simulink model "th_duty_cycle_waveform_generator"  (R2020b)
settings: Solver=FixedStepAuto  StartTime=0.0  StopTime=10.0  FixedStep=6.25e-6  RelTol=1e-3
values from neighbouring files (symbols this model uses):
  parOmodFact = 1.0    [dd_model_under_test_data.sldd]
  th_parOutp1TestTol = 0.01    [dd_test_harness_data.sldd]
  th_parOutp2TestTol = 0.0001    [dd_test_harness_data.sldd]
  th_parPWMMode = 4.0    [dd_test_harness_data.sldd]
  th_parSimModeFlag = 0    [dd_test_harness_data.sldd]
libraries: simulink x2
settings Model: DataDictionary=dd_test_harness_data.sldd  EnableAccessToBaseWorkspace=off  PauseTimes=1  Creator=CAV2OFO  LastModifiedBy=CAV2OFO
settings DebuggingCC: ParameterPrecisionLossMsg=none

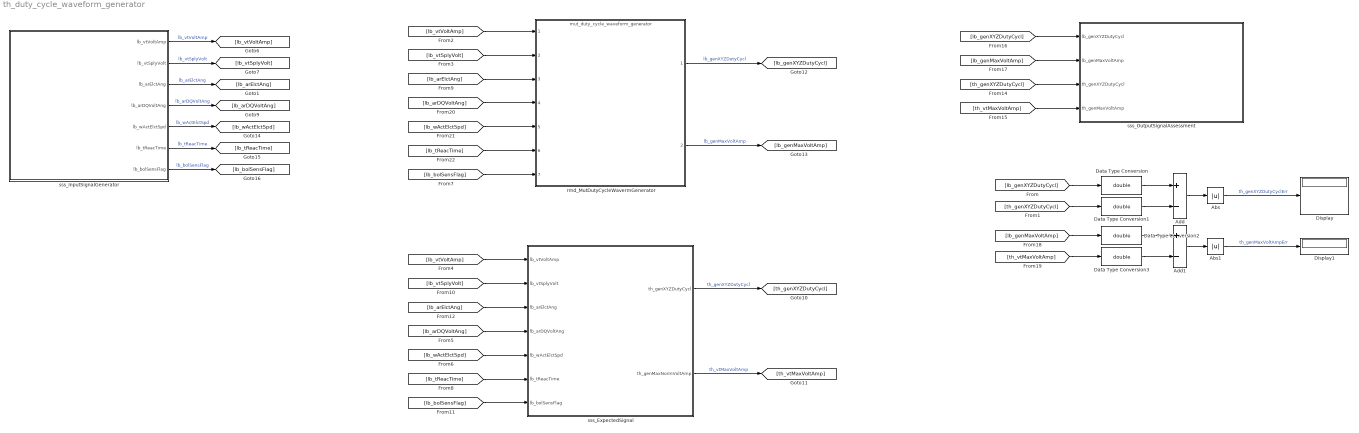
== system th_duty_cycle_waveform_generator ==
  Abs : Abs
  Abs1 : Abs
  Add : Sum  Inputs=+-  OutDataTypeStr=double
  Add1 : Sum  Inputs=+-  OutDataTypeStr=double
  Data Type Conversion{,1..3} (4 alike) : DataTypeConversion  OutDataTypeStr=double
  Display : Display
  Display1 : Display
  rmd_MutDutyCycleWavermGenerator : ModelReference  ModelNameDialog=mut_duty_cycle_waveform_generator  SimulationMode=Normal  ModelReferenceVersion=1.54
  sss_ExpectedSignal : Subsystem
  sss_InputSignalGenerator : Subsystem  InitFcn=|
      | Simulink.suppressDiagnostic([gcb,'/Data Type Conversion1'],...
      |  'SimulinkFixedPoint:util:Overflowoccurred');
      | Simulink.suppressDiagnostic([gcb,'/Data Type Conversion2'],...
      |  'SimulinkFixedPoint:util:Overflowoccurred');
  sss_OutputSignalAssessment : Subsystem
  wires:
  rmd_MutDutyCycleWavermGenerator/1 -> [lb_genXYZDutyCycl]  "lb_genXYZDutyCycl"
  rmd_MutDutyCycleWavermGenerator/2 -> [lb_genMaxVoltAmp]  "lb_genMaxVoltAmp"
  sss_ExpectedSignal/1(th_genXYZDutyCycl) -> [th_genXYZDutyCycl]  "th_genXYZDutyCycl"
  [lb_genXYZDutyCycl] -> Data Type Conversion/1
  [th_genXYZDutyCycl] -> Data Type Conversion1/1
  [lb_genXYZDutyCycl] -> sss_OutputSignalAssessment/1(lb_genXYZDutyCycl)
  Add1/1 -> Abs1/1
  Add/1 -> Abs/1
  Data Type Conversion1/1 -> Add/2
  Data Type Conversion3/1 -> Add1/2
  [th_genXYZDutyCycl] -> sss_OutputSignalAssessment/3(th_genXYZDutyCycl)
  [th_vtMaxVoltAmp] -> sss_OutputSignalAssessment/4(th_genMaxVoltAmp)
  sss_ExpectedSignal/2(th_genMaxNormVoltAmp) -> [th_vtMaxVoltAmp]  "th_vtMaxVoltAmp"
  [th_vtMaxVoltAmp] -> Data Type Conversion3/1
  Data Type Conversion/1 -> Add/1
  Data Type Conversion2/1 -> Add1/1
  Abs1/1 -> Display1/1  "th_genMaxVoltAmpErr"
  [lb_genMaxVoltAmp] -> sss_OutputSignalAssessment/2(lb_genMaxVoltAmp)
  [lb_genMaxVoltAmp] -> Data Type Conversion2/1
  Abs/1 -> Display/1  "th_genXYZDutyCyclErr"
  [lb_vtVoltAmp] -> rmd_MutDutyCycleWavermGenerator/1
  [lb_vtSplyVolt] -> rmd_MutDutyCycleWavermGenerator/2
  [lb_arElctAng] -> rmd_MutDutyCycleWavermGenerator/3
  [lb_arDQVoltAng] -> rmd_MutDutyCycleWavermGenerator/4
  [lb_wActElctSpd] -> rmd_MutDutyCycleWavermGenerator/5
  [lb_tReacTime] -> rmd_MutDutyCycleWavermGenerator/6
  [lb_bolSensFlag] -> rmd_MutDutyCycleWavermGenerator/7
  sss_InputSignalGenerator/1(lb_vtVoltAmp) -> [lb_vtVoltAmp]  "lb_vtVoltAmp"
  sss_InputSignalGenerator/2(lb_vtSplyVolt) -> [lb_vtSplyVolt]  "lb_vtSplyVolt"
  sss_InputSignalGenerator/3(lb_arElctAng) -> [lb_arElctAng]  "lb_arElctAng"
  sss_InputSignalGenerator/4(lb_arDQVoltAng) -> [lb_arDQVoltAng]  "lb_arDQVoltAng"
  sss_InputSignalGenerator/5(lb_wActElctSpd) -> [lb_wActElctSpd]  "lb_wActElctSpd"
  sss_InputSignalGenerator/6(lb_tReacTime) -> [lb_tReacTime]  "lb_tReacTime"
  sss_InputSignalGenerator/7(lb_bolSensFlag) -> [lb_bolSensFlag]  "lb_bolSensFlag"
  [lb_vtVoltAmp] -> sss_ExpectedSignal/1(lb_vtVoltAmp)
  [lb_vtSplyVolt] -> sss_ExpectedSignal/2(lb_vtSplyVolt)
  [lb_arElctAng] -> sss_ExpectedSignal/3(lb_arElctAng)
  [lb_arDQVoltAng] -> sss_ExpectedSignal/4(lb_arDQVoltAng)
  [lb_wActElctSpd] -> sss_ExpectedSignal/5(lb_wActElctSpd)
  [lb_tReacTime] -> sss_ExpectedSignal/6(lb_tReacTime)
  [lb_bolSensFlag] -> sss_ExpectedSignal/7(lb_bolSensFlag)

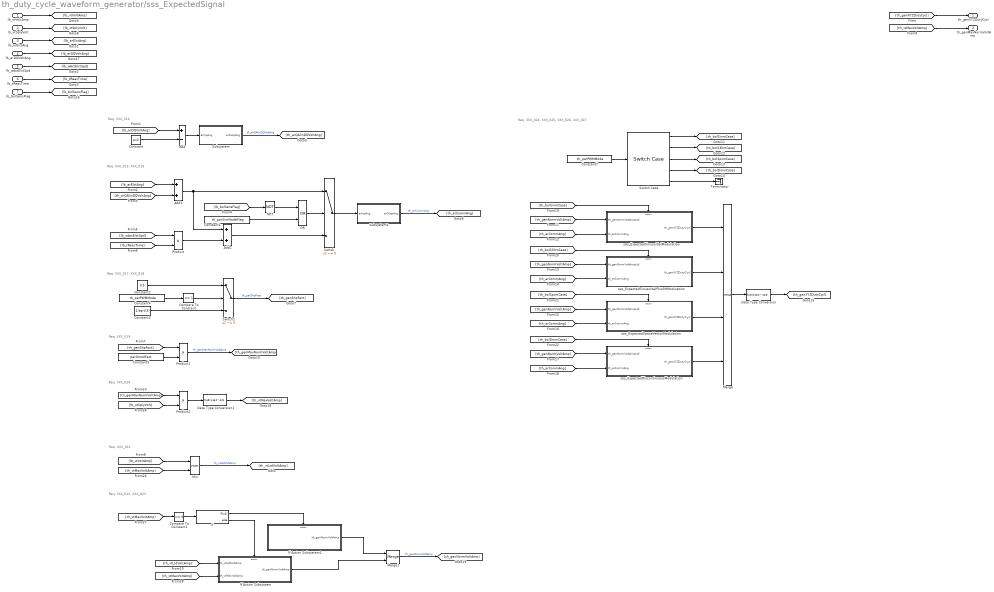
== system th_duty_cycle_waveform_generator/sss_ExpectedSignal ==
  note: Req. XXX_024, XXX_025, XXX_026, XXX_027
  note: Req. XXX_021
  note: Req. XXX_019
  note: Req. XXX_017, XXX_018
  note: Req. XXX_015, XXX_016
  note: Req. XXX_014
  note: Req. XXX_020
  note: Req. XXX_022, XXX_023
  lb_vtVoltAmp : Inport  Interpolate=off
  lb_vtSplyVolt : Inport  Port=2  Interpolate=off
  lb_arElctAng : Inport  Port=3  OutDataTypeStr=fixdt(0,16,pi*2^-15,0)  Interpolate=off
  lb_arDQVoltAng : Inport  Port=4  OutDataTypeStr=fixdt(0,16,pi*2^-15,0)  Interpolate=off
  lb_wActElctSpd : Inport  Port=5  Interpolate=off
  lb_tReacTime : Inport  Port=6  Interpolate=off
  lb_bolSensFlag : Inport  Port=7  OutDataTypeStr=boolean
  Add : Sum  Inputs=+-
  Add1 : Sum
  Add2 : Sum
  Compare To Constant : simulink/Logic and Bit Operations/Compare To Constant  relop===  const=1  OutDataTypeStr=boolean
  Compare To Constant1 : simulink/Logic and Bit Operations/Compare To Constant  relop===  const=0  OutDataTypeStr=boolean
  Constant : Constant  Value=pi/2
  Constant1 : Constant  Value=th_parSimModeFlag
  Constant2 : Constant  Value=0.5
  Constant3 : Constant  Value=1/sqrt(3)
  Constant4 : Constant  Value=th_parPWMMode
  Constant5 : Constant  Value=parOmodFact
  Constant7 : Constant  Value=th_parPWMMode
  Data Type Conversion : DataTypeConversion  OutDataTypeStr=fixdt(0,16,2^-15,0)
  Data Type Conversion1 : DataTypeConversion  OutDataTypeStr=fixdt(1,16,2^-9,0)
  If : If  IfExpression=u1
  If Action Subsystem : Subsystem  TreatAsAtomicUnit=on
  If Action Subsystem1 : Subsystem  TreatAsAtomicUnit=on
  Merge : Merge  Inputs=4
  Merge1 : Merge
  Min : MinMax  Inputs=2
  NOT : Logic  Operator=NOT  IconShape=distinctive  AllPortsSameDT=off  OutDataTypeStr=boolean
  OR : Logic  Operator=OR  AllPortsSameDT=off  OutDataTypeStr=boolean
  Product : Product
  Product1 : Product
  Product2 : Product  OutDataTypeStr=Inherit: Inherit via back propagation
  Subsystem : Subsystem
  Subsystem1 : Subsystem
  Switch : Switch  Criteria=u2 ~= 0
  Switch Case : SwitchCase  CaseConditions={1,2,3,4}
  Switch1 : Switch  Criteria=u2 ~= 0
  Terminator : Terminator
  sas_ExpectedDiscontinuousModulation : Subsystem  TreatAsAtomicUnit=on
  sas_ExpectedSinusoidalModulation : Subsystem  TreatAsAtomicUnit=on
  sas_ExpectedSinusoidalPlus3HModulation : Subsystem  TreatAsAtomicUnit=on
  sas_ExpectedSpaceVectorModulation : Subsystem  TreatAsAtomicUnit=on
  th_genXYZDutyCycl : Outport
  th_genMaxNormVoltAmp : Outport  Port=2
  wires:
  [lb_arDQVoltAng] -> Add/1
  Constant/1 -> Add/2
  Subsystem/1(arOutpAng) -> [th_arQAlinDQVoltAng]  "th_arQAlinDQVoltAng"
  [lb_arElctAng] -> Add1/1
  [th_arQAlinDQVoltAng] -> Add1/2
  Constant1/1 -> OR/2
  OR/1 -> Switch/2
  [lb_bolSensFlag] -> NOT/1
  NOT/1 -> OR/1
  Add1/1 -> Add2/1, Switch/1
  Add2/1 -> Switch/3
  [lb_tReacTime] -> Product/2
  [lb_wActElctSpd] -> Product/1
  Product/1 -> Add2/2
  Switch/1 -> Subsystem1/1(arInpAng)
  Constant4/1 -> Compare To Constant/1
  Compare To Constant/1 -> Switch1/2
  Constant2/1 -> Switch1/1
  Constant3/1 -> Switch1/3
  Switch1/1 -> [th_genShpFact]  "th_parShpFact"
  [th_genShpFact] -> Product1/1
  Constant5/1 -> Product1/2
  Product1/1 -> [th_genMaxNormVoltAmp]  "th_genMaxNormVoltAmp"
  [lb_vtVoltAmp] -> Min/1
  [th_vtMaxVoltAmp] -> Min/2
  Min/1 -> [th_vtLtdVoltAmp]  "th_vtLtdVoltAmp"
  Constant7/1 -> Switch Case/1
  [th_genNormVoltAmp] -> sas_ExpectedSinusoidalModulation/1(th_genNormVoltAmpLtd)
  [th_arCommAng] -> sas_ExpectedSinusoidalModulation/2(th_arCommAng)
  [th_arCommAng] -> sas_ExpectedSinusoidalPlus3HModulation/2(th_arCommAng)
  [th_genNormVoltAmp] -> sas_ExpectedSinusoidalPlus3HModulation/1(th_genNormVoltAmpLtd)
  [th_arCommAng] -> sas_ExpectedSpaceVectorModulation/2(th_arCommAng)
  [th_genNormVoltAmp] -> sas_ExpectedSpaceVectorModulation/1(th_genNormVoltAmpLtd)
  [th_arCommAng] -> sas_ExpectedDiscontinuousModulation/2(th_arCommAng)
  [th_genNormVoltAmp] -> sas_ExpectedDiscontinuousModulation/1(th_genNormVoltAmpLtd)
  Switch Case/5 -> Terminator/1
  Switch Case/1 -> [th_bolSinmCase]
  Switch Case/2 -> [th_bolS3hmCase]
  Switch Case/3 -> [th_bolSpvmCase]
  Switch Case/4 -> [th_bolDmmCase]
  [th_bolSinmCase] -> sas_ExpectedSinusoidalModulation/Action
  [th_bolS3hmCase] -> sas_ExpectedSinusoidalPlus3HModulation/Action
  [th_bolSpvmCase] -> sas_ExpectedSpaceVectorModulation/Action
  [th_bolDmmCase] -> sas_ExpectedDiscontinuousModulation/Action
  sas_ExpectedSinusoidalPlus3HModulation/1(th_genXYZDutyCycl) -> Merge/2
  sas_ExpectedSinusoidalModulation/1(th_genXYZDutyCycl) -> Merge/1
  sas_ExpectedSpaceVectorModulation/1(th_genXYZDutyCycl) -> Merge/3
  sas_ExpectedDiscontinuousModulation/1(th_genXYZDutyCycl) -> Merge/4
  Merge/1 -> Data Type Conversion/1
  [th_genXYZDutyCycl] -> th_genXYZDutyCycl/1
  [th_vtMaxVoltAmp] -> th_genMaxNormVoltAmp/1
  lb_arDQVoltAng/1 -> [lb_arDQVoltAng]
  lb_arElctAng/1 -> [lb_arElctAng]
  lb_vtSplyVolt/1 -> [lb_vtSplyVolt]
  lb_bolSensFlag/1 -> [lb_bolSensFlag]
  lb_tReacTime/1 -> [lb_tReacTime]
  lb_vtVoltAmp/1 -> [lb_vtVoltAmp]
  lb_wActElctSpd/1 -> [lb_wActElctSpd]
  [th_genMaxNormVoltAmp] -> Product2/1
  [lb_vtSplyVolt] -> Product2/2
  Product2/1 -> Data Type Conversion1/1
  Data Type Conversion/1 -> [th_genXYZDutyCycl]
  [th_vtMaxVoltAmp] -> Compare To Constant1/1
  Compare To Constant1/1 -> If/1
  [th_vtLtdVoltAmp] -> If Action Subsystem/1(th_vtLtdVoltAmp)
  [th_vtMaxVoltAmp] -> If Action Subsystem/2(th_vtMaxVoltAmp)
  If/2 -> If Action Subsystem/Action
  If/1 -> If Action Subsystem1/Action
  Merge1/1 -> [th_genNormVoltAmp]  "th_genNormVoltAmp"
  If Action Subsystem1/1(th_genNormVoltAmp) -> Merge1/1
  If Action Subsystem/1(th_genNormVoltAmp) -> Merge1/2
  Data Type Conversion1/1 -> [th_vtMaxVoltAmp]
  Add/1 -> Subsystem/1(arInpAng)
  Subsystem1/1(arOutpAng) -> [th_arCommAng]  "th_arCommAng"

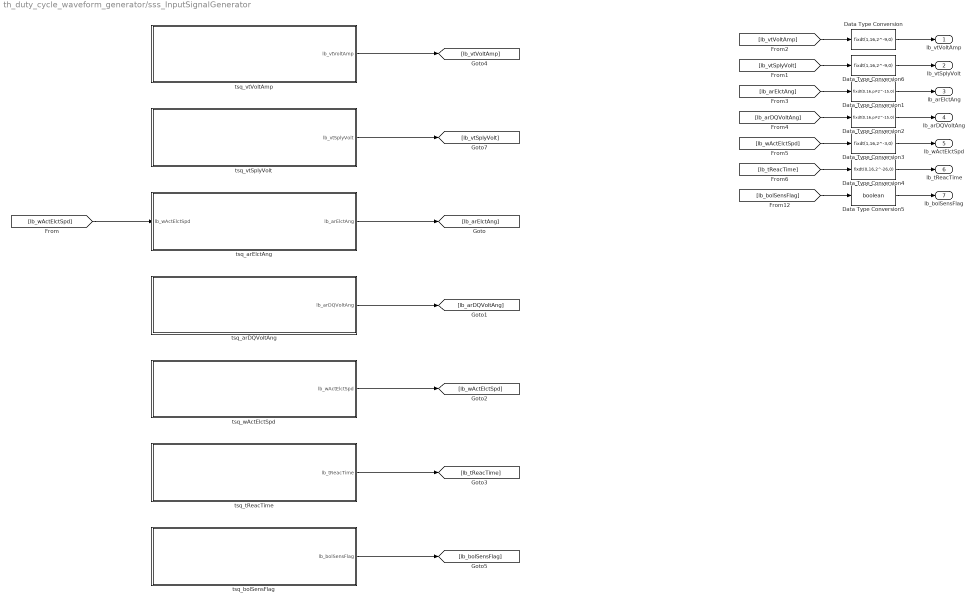
== system th_duty_cycle_waveform_generator/sss_InputSignalGenerator ==
  Data Type Conversion : DataTypeConversion  OutDataTypeStr=fixdt(1,16,2^-9,0)
  Data Type Conversion1 : DataTypeConversion  OutDataTypeStr=fixdt(0,16,pi*2^-15,0)
  Data Type Conversion2 : DataTypeConversion  OutDataTypeStr=fixdt(0,16,pi*2^-15,0)
  Data Type Conversion3 : DataTypeConversion  OutDataTypeStr=fixdt(1,16,2^-3,0)
  Data Type Conversion4 : DataTypeConversion  OutDataTypeStr=fixdt(0,16,2^-26,0)
  Data Type Conversion5 : DataTypeConversion  OutDataTypeStr=boolean
  Data Type Conversion6 : DataTypeConversion  OutDataTypeStr=fixdt(1,16,2^-9,0)
  tsq_arDQVoltAng : Test Sequence  TreatAsAtomicUnit=on
  tsq_arElctAng : Test Sequence  TreatAsAtomicUnit=on
  tsq_bolSensFlag : Test Sequence  TreatAsAtomicUnit=on
  tsq_tReacTime : Test Sequence  TreatAsAtomicUnit=on
  tsq_vtSplyVolt : Test Sequence  TreatAsAtomicUnit=on
  tsq_vtVoltAmp : Test Sequence  TreatAsAtomicUnit=on
  tsq_wActElctSpd : Test Sequence  TreatAsAtomicUnit=on
  lb_vtVoltAmp : Outport
  lb_vtSplyVolt : Outport  Port=2
  lb_arElctAng : Outport  Port=3
  lb_arDQVoltAng : Outport  Port=4
  lb_wActElctSpd : Outport  Port=5
  lb_tReacTime : Outport  Port=6
  lb_bolSensFlag : Outport  Port=7
  wires:
  [lb_arElctAng] -> Data Type Conversion1/1
  [lb_vtVoltAmp] -> Data Type Conversion/1
  [lb_arDQVoltAng] -> Data Type Conversion2/1
  [lb_wActElctSpd] -> Data Type Conversion3/1
  [lb_tReacTime] -> Data Type Conversion4/1
  tsq_vtVoltAmp/1(lb_vtVoltAmp) -> [lb_vtVoltAmp]
  tsq_arElctAng/1(lb_arElctAng) -> [lb_arElctAng]
  tsq_arDQVoltAng/1(lb_arDQVoltAng) -> [lb_arDQVoltAng]
  tsq_wActElctSpd/1(lb_wActElctSpd) -> [lb_wActElctSpd]
  tsq_tReacTime/1(lb_tReacTime) -> [lb_tReacTime]
  tsq_bolSensFlag/1(lb_bolSensFlag) -> [lb_bolSensFlag]
  Data Type Conversion/1 -> lb_vtVoltAmp/1
  Data Type Conversion1/1 -> lb_arElctAng/1
  Data Type Conversion2/1 -> lb_arDQVoltAng/1
  Data Type Conversion3/1 -> lb_wActElctSpd/1
  Data Type Conversion4/1 -> lb_tReacTime/1
  [lb_bolSensFlag] -> Data Type Conversion5/1
  Data Type Conversion5/1 -> lb_bolSensFlag/1
  [lb_wActElctSpd] -> tsq_arElctAng/1(lb_wActElctSpd)
  Data Type Conversion6/1 -> lb_vtSplyVolt/1
  [lb_vtSplyVolt] -> Data Type Conversion6/1
  tsq_vtSplyVolt/1(lb_vtSplyVolt) -> [lb_vtSplyVolt]

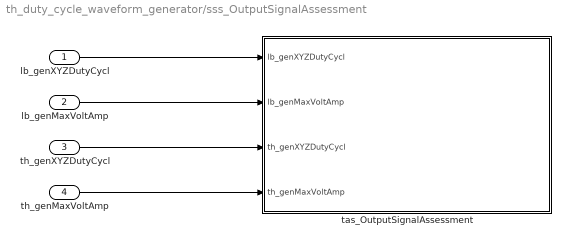
== system th_duty_cycle_waveform_generator/sss_OutputSignalAssessment ==
  lb_genXYZDutyCycl : Inport
  lb_genMaxVoltAmp : Inport  Port=2
  th_genXYZDutyCycl : Inport  Port=3
  th_genMaxVoltAmp : Inport  Port=4
  tas_OutputSignalAssessment : Test Sequence  TreatAsAtomicUnit=on
  wires:
  lb_genXYZDutyCycl/1 -> tas_OutputSignalAssessment/1(lb_genXYZDutyCycl)
  lb_genMaxVoltAmp/1 -> tas_OutputSignalAssessment/2(lb_genMaxVoltAmp)
  th_genXYZDutyCycl/1 -> tas_OutputSignalAssessment/3(th_genXYZDutyCycl)
  th_genMaxVoltAmp/1 -> tas_OutputSignalAssessment/4(th_genMaxVoltAmp)

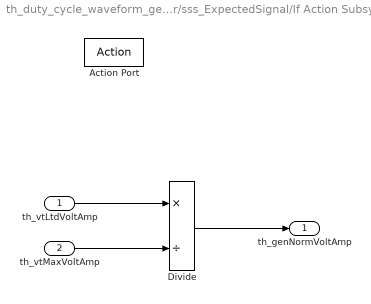
== system th_duty_cycle_waveform_generator/sss_ExpectedSignal/If Action Subsystem ==
  th_vtLtdVoltAmp : Inport
  th_vtMaxVoltAmp : Inport  Port=2
  Action Port : ActionPort  ActionPortLabel=else
  Divide : Product  Inputs=*/  OutDataTypeStr=double
  th_genNormVoltAmp : Outport
  wires:
  th_vtLtdVoltAmp/1 -> Divide/1
  th_vtMaxVoltAmp/1 -> Divide/2
  Divide/1 -> th_genNormVoltAmp/1

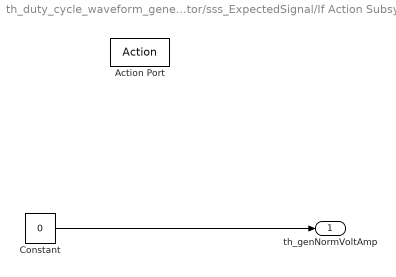
== system th_duty_cycle_waveform_generator/sss_ExpectedSignal/If Action Subsystem1 ==
  Action Port : ActionPort  ActionPortLabel=if(u1)
  Constant : Constant  Value=0  OutDataTypeStr=double
  th_genNormVoltAmp : Outport
  wires:
  Constant/1 -> th_genNormVoltAmp/1

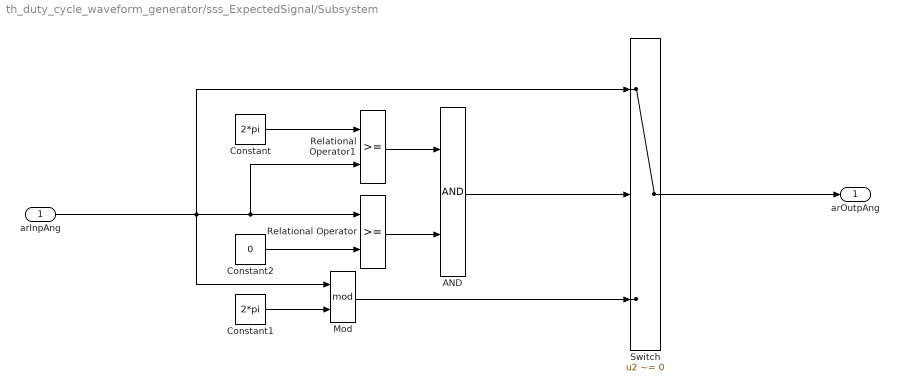
== system th_duty_cycle_waveform_generator/sss_ExpectedSignal/Subsystem ==
  arInpAng : Inport
  AND : Logic  AllPortsSameDT=off  OutDataTypeStr=boolean
  Constant : Constant  Value=2*pi  OutDataTypeStr=Inherit: Inherit via back propagation
  Constant1 : Constant  Value=2*pi  OutDataTypeStr=Inherit: Inherit via back propagation
  Constant2 : Constant  Value=0  OutDataTypeStr=Inherit: Inherit via back propagation
  Mod : Math  Operator=mod  SaturateOnIntegerOverflow=on
  Relational Operator : RelationalOperator  OutDataTypeStr=boolean  RndMeth=Simplest
  Relational Operator1 : RelationalOperator  OutDataTypeStr=boolean  RndMeth=Simplest
  Switch : Switch  Criteria=u2 ~= 0
  arOutpAng : Outport
  wires:
  Constant/1 -> Relational Operator1/1
  arInpAng/1 -> Mod/1, Switch/1, Relational Operator/1, Relational Operator1/2
  Constant2/1 -> Relational Operator/2
  Relational Operator1/1 -> AND/1
  Relational Operator/1 -> AND/2
  AND/1 -> Switch/2
  Constant1/1 -> Mod/2
  Mod/1 -> Switch/3
  Switch/1 -> arOutpAng/1

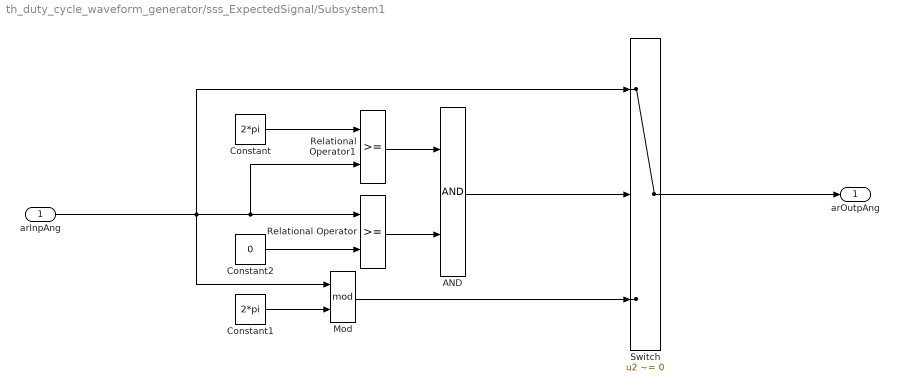
== system th_duty_cycle_waveform_generator/sss_ExpectedSignal/Subsystem1 ==
  arInpAng : Inport
  AND : Logic  AllPortsSameDT=off  OutDataTypeStr=boolean
  Constant : Constant  Value=2*pi  OutDataTypeStr=Inherit: Inherit via back propagation
  Constant1 : Constant  Value=2*pi  OutDataTypeStr=Inherit: Inherit via back propagation
  Constant2 : Constant  Value=0  OutDataTypeStr=Inherit: Inherit via back propagation
  Mod : Math  Operator=mod  SaturateOnIntegerOverflow=on
  Relational Operator : RelationalOperator  OutDataTypeStr=boolean  RndMeth=Simplest
  Relational Operator1 : RelationalOperator  OutDataTypeStr=boolean  RndMeth=Simplest
  Switch : Switch  Criteria=u2 ~= 0
  arOutpAng : Outport
  wires:
  Constant/1 -> Relational Operator1/1
  arInpAng/1 -> Mod/1, Switch/1, Relational Operator/1, Relational Operator1/2
  Constant2/1 -> Relational Operator/2
  Relational Operator1/1 -> AND/1
  Relational Operator/1 -> AND/2
  AND/1 -> Switch/2
  Constant1/1 -> Mod/2
  Mod/1 -> Switch/3
  Switch/1 -> arOutpAng/1

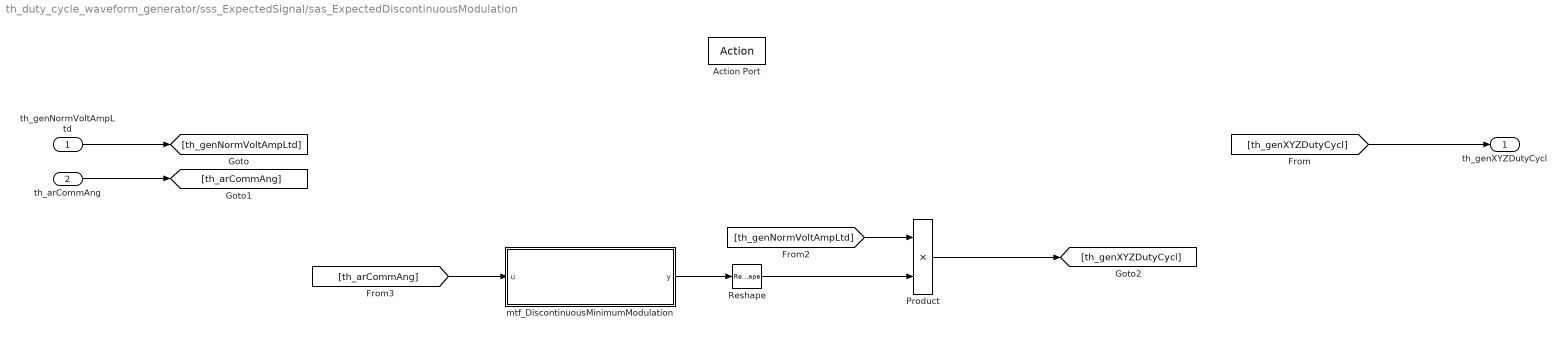
== system th_duty_cycle_waveform_generator/sss_ExpectedSignal/sas_ExpectedDiscontinuousModulation ==
  th_genNormVoltAmpLtd : Inport
  th_arCommAng : Inport  Port=2
  Action Port : ActionPort  ActionPortLabel=case [ 4 ]:
  Product : Product
  Reshape : Reshape
  mtf_DiscontinuousMinimumModulation : MATLAB Function  TreatAsAtomicUnit=on
  th_genXYZDutyCycl : Outport
  wires:
  [th_genXYZDutyCycl] -> th_genXYZDutyCycl/1
  th_genNormVoltAmpLtd/1 -> [th_genNormVoltAmpLtd]
  th_arCommAng/1 -> [th_arCommAng]
  [th_genNormVoltAmpLtd] -> Product/1
  Product/1 -> [th_genXYZDutyCycl]
  mtf_DiscontinuousMinimumModulation/1(y) -> Reshape/1
  [th_arCommAng] -> mtf_DiscontinuousMinimumModulation/1(u)
  Reshape/1 -> Product/2

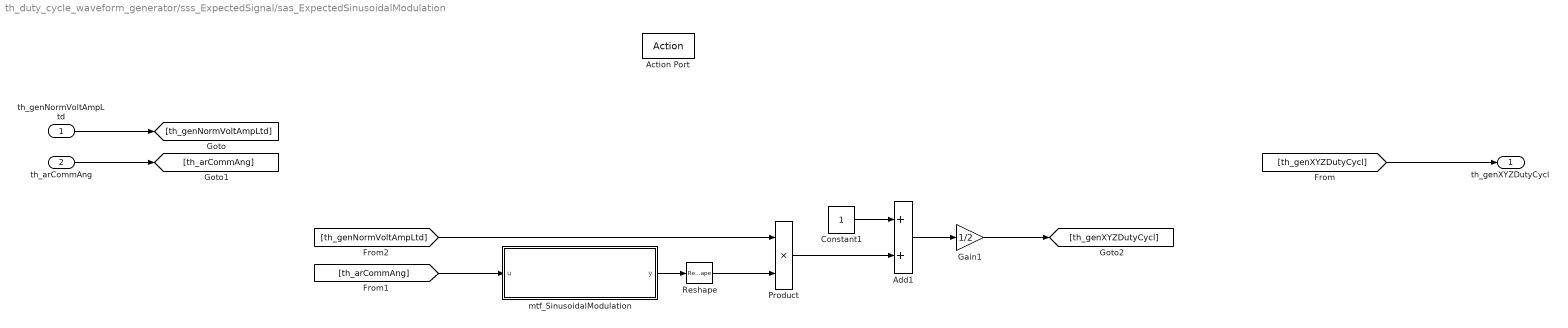
== system th_duty_cycle_waveform_generator/sss_ExpectedSignal/sas_ExpectedSinusoidalModulation ==
  th_genNormVoltAmpLtd : Inport
  th_arCommAng : Inport  Port=2
  Action Port : ActionPort  ActionPortLabel=case [ 1 ]:
  Add1 : Sum
  Constant1 : Constant
  Gain1 : Gain  Gain=1/2
  Product : Product
  Reshape : Reshape
  mtf_SinusoidalModulation : MATLAB Function  TreatAsAtomicUnit=on
  th_genXYZDutyCycl : Outport
  wires:
  [th_genXYZDutyCycl] -> th_genXYZDutyCycl/1
  th_genNormVoltAmpLtd/1 -> [th_genNormVoltAmpLtd]
  th_arCommAng/1 -> [th_arCommAng]
  [th_arCommAng] -> mtf_SinusoidalModulation/1(u)
  mtf_SinusoidalModulation/1(y) -> Reshape/1
  [th_genNormVoltAmpLtd] -> Product/1
  Product/1 -> Add1/2
  Constant1/1 -> Add1/1
  Add1/1 -> Gain1/1
  Gain1/1 -> [th_genXYZDutyCycl]
  Reshape/1 -> Product/2

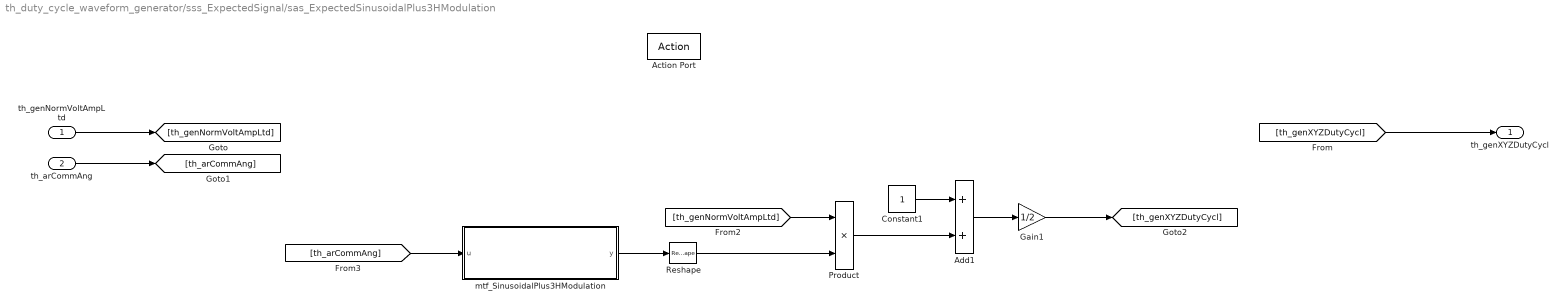
== system th_duty_cycle_waveform_generator/sss_ExpectedSignal/sas_ExpectedSinusoidalPlus3HModulation ==
  th_genNormVoltAmpLtd : Inport
  th_arCommAng : Inport  Port=2
  Action Port : ActionPort  ActionPortLabel=case [ 2 ]:
  Add1 : Sum
  Constant1 : Constant
  Gain1 : Gain  Gain=1/2
  Product : Product
  Reshape : Reshape
  mtf_SinusoidalPlus3HModulation : MATLAB Function  TreatAsAtomicUnit=on
  th_genXYZDutyCycl : Outport
  wires:
  [th_genXYZDutyCycl] -> th_genXYZDutyCycl/1
  th_genNormVoltAmpLtd/1 -> [th_genNormVoltAmpLtd]
  th_arCommAng/1 -> [th_arCommAng]
  [th_genNormVoltAmpLtd] -> Product/1
  Product/1 -> Add1/2
  Constant1/1 -> Add1/1
  Add1/1 -> Gain1/1
  Gain1/1 -> [th_genXYZDutyCycl]
  mtf_SinusoidalPlus3HModulation/1(y) -> Reshape/1
  [th_arCommAng] -> mtf_SinusoidalPlus3HModulation/1(u)
  Reshape/1 -> Product/2

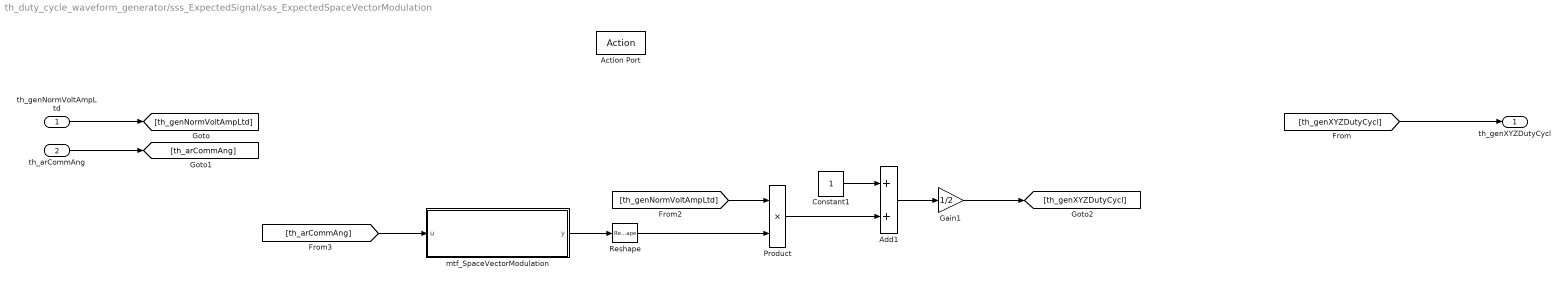
== system th_duty_cycle_waveform_generator/sss_ExpectedSignal/sas_ExpectedSpaceVectorModulation ==
  th_genNormVoltAmpLtd : Inport
  th_arCommAng : Inport  Port=2
  Action Port : ActionPort  ActionPortLabel=case [ 3 ]:
  Add1 : Sum
  Constant1 : Constant
  Gain1 : Gain  Gain=1/2
  Product : Product
  Reshape : Reshape
  mtf_SpaceVectorModulation : MATLAB Function  TreatAsAtomicUnit=on
  th_genXYZDutyCycl : Outport
  wires:
  [th_genXYZDutyCycl] -> th_genXYZDutyCycl/1
  th_genNormVoltAmpLtd/1 -> [th_genNormVoltAmpLtd]
  th_arCommAng/1 -> [th_arCommAng]
  [th_genNormVoltAmpLtd] -> Product/1
  Product/1 -> Add1/2
  Constant1/1 -> Add1/1
  Add1/1 -> Gain1/1
  Gain1/1 -> [th_genXYZDutyCycl]
  mtf_SpaceVectorModulation/1(y) -> Reshape/1
  [th_arCommAng] -> mtf_SpaceVectorModulation/1(u)
  Reshape/1 -> Product/2

== stateflow chart th_duty_cycle_waveform_generator/sss_OutputSignalAssessment/tas_OutputSignalAssessment ==
  settings: stateMachineType=SIMPLIFIED_MACHINE
  state verify
    error1 = abs(double(lb_genXYZDutyCycl)-double(th_genXYZDutyCycl));
    error2 = abs(double(lb_genMaxVoltAmp)-double(th_genMaxVoltAmp));
    verify(all(error1 <= th_parOutp1TestTol),'The actual and expected XYZ duty cycles output match');
    verify(error2 <= th_parOutp2TestTol,'The actual and expected maximum voltage amplitude output match');
  (default) -> verify
  data: lb_genXYZDutyCycl input fixdt(0,16,2^-15,0) size=3; lb_genMaxVoltAmp input fixdt(1,16,2^-9,0); th_parOutp1TestTol parameter; error1 local double size=3; th_genXYZDutyCycl input fixdt(0,16,2^-15,0) size=3; th_genMaxVoltAmp input fixdt(1,16,2^-9,0); th_parOutp2TestTol parameter; error2 local

== stateflow chart th_duty_cycle_waveform_generator/sss_InputSignalGenerator/tsq_arElctAng ==
  settings: stateMachineType=SIMPLIFIED_MACHINE
  state Scenario_1
    state Init
      lb_arElctAng = 0;
    state step_1
      lb_arElctAng = lb_wActElctSpd*et;
    (default) -> Init
    Init -> step_1 : [
        | true
        | ]
  (default) -> Scenario_1 : {assert(th_parTestProcElctAngIndx == 1,'The value of Scenario Parameter ''th_parTestProcElctAngIndx'' is not valid. Use the index of the scenario to specify it.')}
  data: lb_arElctAng output; th_parTestProcElctAngIndx parameter =1; lb_wActElctSpd input

== stateflow chart th_duty_cycle_waveform_generator/sss_InputSignalGenerator/tsq_arDQVoltAng ==
  settings: stateMachineType=SIMPLIFIED_MACHINE
  state Scenario_1
    state Init
      lb_arDQVoltAng = pi;
    (default) -> Scenario_1.Init
  state Scenario_2
    state Init
      lb_arDQVoltAng = 0;
    state Increase_1
      if et == 0
      lb_arDQVoltAng = lb_arDQVoltAng + pi*2^(-15);
      end
    state Wait_1
    state Wait_2
    Increase_1 -> (junction 81) [order 1] : [
        | lb_arDQVoltAng > 2*pi
        | ]
    (default) -> Scenario_2.Init
    Scenario_2.Init -> Increase_1 : [
        | after(2,tick)
        | ]
    Increase_1 -> Wait_1 [order 2] : [
        | after(1,tick)
        | ]
    Wait_1 -> Increase_1 : [
        | after(1,tick)
        | ]
    (junction 79) -> Wait_2
    (junction 81) -> (junction 79)
  (default) -> Scenario_1 [order 1] : [th_parTestProcDQVoltAngIndx == 1]
  (default) -> Scenario_2 [order 2] : {assert(th_parTestProcDQVoltAngIndx == 2,'The value of Scenario Parameter ''th_parTestProcDQVoltAngIndx'' is not valid. Use the index of the scenario to specify it.')}
  data: lb_arDQVoltAng output; th_parTestProcDQVoltAngIndx parameter =2

== matlab function th_duty_cycle_waveform_generator/sss_ExpectedSignal/sas_ExpectedSinusoidalPlus3HModulation/mtf_SinusoidalPlus3HModulation ==
  data: u input; y output
function y = fcn(u)

f = @(t) -sin(t)-1/6*sin(3*t);

u_vect = linspace(0,2*pi,1000);

y = [f(u)/max(abs(f(u_vect))), ...
    f(u-2/3*pi)/max(abs(f(u_vect-2/3*pi))),...
    f(u-4/3*pi)/max(abs(f(u_vect-4/3*pi)))];

end

== stateflow chart th_duty_cycle_waveform_generator/sss_InputSignalGenerator/tsq_wActElctSpd ==
  settings: stateMachineType=SIMPLIFIED_MACHINE
  state Scenario_1
    state Init
      lb_wActElctSpd = 3000*5*pi/30;;
    (default) -> Init
  (default) -> Scenario_1 : {assert(th_parTestProcActElctSpdIndx == 1,'The value of Scenario Parameter ''th_parTestProcActElctSpdIndx'' is not valid. Use the index of the scenario to specify it.')}
  data: lb_wActElctSpd output; th_parTestProcActElctSpdIndx parameter =1

== stateflow chart th_duty_cycle_waveform_generator/sss_InputSignalGenerator/tsq_bolSensFlag ==
  settings: stateMachineType=SIMPLIFIED_MACHINE
  state Scenario_1
    state Init
      lb_bolSensFlag = true;
    (default) -> Init
  (default) -> Scenario_1 : {assert(th_parTestProcSensFlagIndx == 1,'The value of Scenario Parameter ''th_parTestProcSensFlagIndx'' is not valid. Use the index of the scenario to specify it.')}
  data: lb_bolSensFlag output; th_parTestProcSensFlagIndx parameter =1

== stateflow chart th_duty_cycle_waveform_generator/sss_InputSignalGenerator/tsq_tReacTime ==
  settings: stateMachineType=SIMPLIFIED_MACHINE
  state Scenario_1
    state Init
      lb_tReacTime = 62.5e-6;
    (default) -> Init
  (default) -> Scenario_1 : {assert(th_parTestProcReacTimeIndx == 1,'The value of Scenario Parameter ''th_parTestProcReacTimeIndx'' is not valid. Use the index of the scenario to specify it.')}
  data: lb_tReacTime output; th_parTestProcReacTimeIndx parameter =1

== stateflow chart th_duty_cycle_waveform_generator/sss_InputSignalGenerator/tsq_vtVoltAmp ==
  settings: stateMachineType=SIMPLIFIED_MACHINE
  state Scenario_1
    state Init
      lb_vtVoltAmp = 0;
    state Step_1
      lb_vtVoltAmp = 6*(0.5*sin(2*pi/2*et)+0.5);
    (default) -> Scenario_1.Init
    Scenario_1.Init -> Scenario_1.Step_1 : [
        | true
        | ]
  state Scenario_2
    state Init
      lb_vtVoltAmp = 0;
    state Step_1
      lb_vtVoltAmp = 2*(0.5*sin(2*pi/2*et)+0.5);
    (default) -> Scenario_2.Init
    Scenario_2.Init -> Scenario_2.Step_1 : [
        | true
        | ]
  (default) -> Scenario_1 [order 1] : [th_parTestProcVoltAmpIndx == 1]
  (default) -> Scenario_2 [order 2] : {assert(th_parTestProcVoltAmpIndx == 2,'The value of Scenario Parameter ''th_parTestProcVoltAmpIndx'' is not valid. Use the index of the scenario to specify it.')}
  data: lb_vtVoltAmp output double; th_parTestProcVoltAmpIndx parameter =2

== matlab function th_duty_cycle_waveform_generator/sss_ExpectedSignal/sas_ExpectedSinusoidalModulation/mtf_SinusoidalModulation ==
  data: u input; y output
function y = fcn(u)

f = @(t) -sin(t);

y = [f(u), ...
    f(u-2/3*pi),...
    f(u-4/3*pi)];

end

== matlab function th_duty_cycle_waveform_generator/sss_ExpectedSignal/sas_ExpectedSpaceVectorModulation/mtf_SpaceVectorModulation ==
  data: u input; y output
function y = fcn(u)

u_vect = linspace(0,2*pi,1000);
fun_1 = @(t) -sin(t);
fun_2 = @(t) -sin(t-2/3*pi);
fun_3 = @(t) -sin(t-4/3*pi);
spv_fun_1 = fun_1(u)-1/2*(max([fun_1(u);fun_2(u);fun_3(u)],[],1)...
    +min([fun_1(u);fun_2(u);fun_3(u)],[],1));
max_spv_fun_1 = max(abs(fun_1(u_vect)-1/2*(max([fun_1(u_vect);fun_2(u_vect);fun_3(u_vect)],[],1)...
    +min([fun_1(u_vect);fun_2(u_vect);fun_3(u_vect)],[],1))));
spv_fun_2 = fun_2(u)-1/2*(max([fun_1(u);fun_2(u);fun_3(u)],[],1)...
    +min([fun_1(u);fun_2(u);fun_3(u)],[],1));
max_spv_fun_2 = max(abs(fun_2(u_vect)-1/2*(max([fun_1(u_vect);fun_2(u_vect);fun_3(u_vect)],[],1)...
    +min([fun_1(u_vect);fun_2(u_vect);fun_3(u_vect)],[],1))));
spv_fun_3 = fun_3(u)-1/2*(max([fun_1(u);fun_2(u);fun_3(u)],[],1)...
    +min([fun_1(u);fun_2(u);fun_3(u)],[],1));
max_spv_fun_3 = max(abs(fun_3(u_vect)-1/2*(max([fun_1(u_vect);fun_2(u_vect);fun_3(u_vect)],[],1)...
    +min([fun_1(u_vect);fun_2(u_vect);fun_3(u_vect)],[],1))));

y = [spv_fun_1/max_spv_fun_1;...
    spv_fun_2/max_spv_fun_2;...
    spv_fun_3/max_spv_fun_3];

end

== matlab function th_duty_cycle_waveform_generator/sss_ExpectedSignal/sas_ExpectedDiscontinuousModulation/mtf_DiscontinuousMinimumModulation ==
  data: u input; y output size=[3 1]
function y = fcn(u)

u_vect = linspace(0,2*pi,1000);
fun_1 = @(t) -sin(t);
fun_2 = @(t) -sin(t-2/3*pi);
fun_3 = @(t) -sin(t-4/3*pi);
dm_fun_1 = fun_1(u)-min([fun_1(u);fun_2(u);fun_3(u)],[],1);
max_dm_fun_1 = max(abs(fun_1(u_vect)-min([fun_1(u_vect);fun_2(u_vect);fun_3(u_vect)],[],1)));
dm_fun_2 = fun_2(u)-min([fun_1(u);fun_2(u);fun_3(u)],[],1);
max_dm_fun_2 = max(abs(fun_2(u_vect)-min([fun_1(u_vect);fun_2(u_vect);fun_3(u_vect)],[],1)));
dm_fun_3 = fun_3(u)-min([fun_1(u);fun_2(u);fun_3(u)],[],1);
max_dm_fun_3 = max(abs(fun_3(u_vect)-min([fun_1(u_vect);fun_2(u_vect);fun_3(u_vect)],[],1)));

y = [dm_fun_1/max_dm_fun_1;...
    dm_fun_2/max_dm_fun_2;...
    dm_fun_3/max_dm_fun_3];

end

== stateflow chart th_duty_cycle_waveform_generator/sss_InputSignalGenerator/tsq_vtSplyVolt ==
  settings: stateMachineType=SIMPLIFIED_MACHINE
  state Scenario_1
    state Init
      lb_vtSplyVolt = 12;
    (default) -> Init
  (default) -> Scenario_1 : {assert(th_parTestProcSplyVoltIndx == 1,'The value of Scenario Parameter ''th_parTestProcSplyVoltIndx'' is not valid. Use the index of the scenario to specify it.')}
  data: lb_vtSplyVolt output double; th_parTestProcSplyVoltIndx parameter =1
